simulink model "DZ1_2c"  (Simulink 7.5)
settings: Solver=ode45  StartTime=0.0  StopTime=100000  RelTol=1e-3
libraries: simulink x1
settings Model: Creator=Hrvoje  LastModifiedBy=Hrvoje

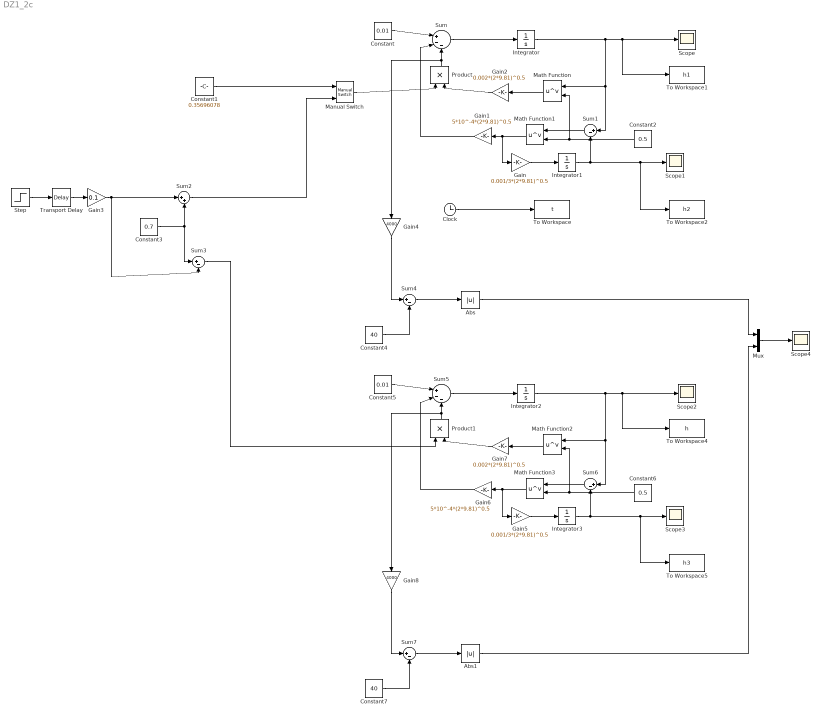
== system DZ1_2c ==
  Abs : Abs  OutDataType=fixdt(1, 16)  OutScaling=2^0
  Abs1 : Abs  OutDataType=fixdt(1, 16)  OutScaling=2^0
  Clock : Clock
      settings: Decimation=10
  Constant : Constant  Value=0.01  OutDataType=fixdt(1, 16)  OutScaling=2^0
  Constant1 : Constant  Value=0.35696078  OutDataType=fixdt(1, 16)  OutScaling=2^0
  Constant2 : Constant  Value=0.5  OutDataType=fixdt(1, 16)  OutScaling=2^0
  Constant3 : Constant  Value=0.7  OutDataType=fixdt(1, 16)  OutScaling=2^0
  Constant4 : Constant  Value=40  OutDataType=fixdt(1, 16)  OutScaling=2^0
  Constant5 : Constant  Value=0.01  OutDataType=fixdt(1, 16)  OutScaling=2^0
  Constant6 : Constant  Value=0.5  OutDataType=fixdt(1, 16)  OutScaling=2^0
  Constant7 : Constant  Value=40  OutDataType=fixdt(1, 16)  OutScaling=2^0
  Gain : Gain  Gain=0.001/3*(2*9.81)^0.5  ParameterDataType=fixdt(1, 16)  ParameterScaling=2^0  OutDataType=fixdt(1, 16)  OutScaling=2^0
  Gain1 : Gain  Gain=5*10^-4*(2*9.81)^0.5  ParameterDataType=fixdt(1, 16)  ParameterScaling=2^0  OutDataType=fixdt(1, 16)  OutScaling=2^0
  Gain2 : Gain  Gain=0.002*(2*9.81)^0.5  ParameterDataType=fixdt(1, 16)  ParameterScaling=2^0  OutDataType=fixdt(1, 16)  OutScaling=2^0
  Gain3 : Gain  Gain=0.1  ParameterDataType=fixdt(1, 16)  ParameterScaling=2^0  OutDataType=fixdt(1, 16)  OutScaling=2^0
  Gain4 : Gain  Gain=4000  ParameterDataType=fixdt(1, 16)  ParameterScaling=2^0  OutDataType=fixdt(1, 16)  OutScaling=2^0
  Gain5 : Gain  Gain=0.001/3*(2*9.81)^0.5  ParameterDataType=fixdt(1, 16)  ParameterScaling=2^0  OutDataType=fixdt(1, 16)  OutScaling=2^0
  Gain6 : Gain  Gain=5*10^-4*(2*9.81)^0.5  ParameterDataType=fixdt(1, 16)  ParameterScaling=2^0  OutDataType=fixdt(1, 16)  OutScaling=2^0
  Gain7 : Gain  Gain=0.002*(2*9.81)^0.5  ParameterDataType=fixdt(1, 16)  ParameterScaling=2^0  OutDataType=fixdt(1, 16)  OutScaling=2^0
  Gain8 : Gain  Gain=4000  ParameterDataType=fixdt(1, 16)  ParameterScaling=2^0  OutDataType=fixdt(1, 16)  OutScaling=2^0
  Integrator{,1..3} (4 alike) : Integrator  InitialCondition=2.6
  Manual Switch : simulink/Signal Routing/Manual Switch  SystemSampleTime=-1  sw=0  action=0  varsize=off
  Math Function{,1..3} (4 alike) : Math  Operator=pow  OutDataType=fixdt(1, 16)  OutScaling=2^0  SaturateOnIntegerOverflow=on
  Mux : Mux  Inputs=2
  Product : Product  OutDataType=fixdt(1, 16)  OutScaling=2^0  RndMeth=Zero
  Product1 : Product  OutDataType=fixdt(1, 16)  OutScaling=2^0  RndMeth=Zero
  Scope{,1..4} (5 alike) : Scope
      Scope2 settings: SaveName=ScopeData4
      Scope3 settings: SaveName=ScopeData5
      Scope4 settings: SaveName=ScopeData2
  Step : Step  SampleTime=0
  Sum : Sum  Inputs=|+--  OutDataType=fixdt(1, 16)  OutScaling=2^0
  Sum{1,3..4,6..7} (5 alike) : Sum  Inputs=|+-  OutDataType=fixdt(1, 16)  OutScaling=2^0
  Sum2 : Sum  Inputs=|++  OutDataType=fixdt(1, 16)  OutScaling=2^0
  Sum5 : Sum  Inputs=|+--  OutDataType=fixdt(1, 16)  OutScaling=2^0
  To Workspace : ToWorkspace  VariableName=t  SampleTime=-1  SaveFormat=Structure
  To Workspace1 : ToWorkspace  VariableName=h1  SampleTime=-1  SaveFormat=Structure
  To Workspace2 : ToWorkspace  VariableName=h2  SampleTime=-1  SaveFormat=Structure
  To Workspace4 : ToWorkspace  VariableName=h  SampleTime=-1  SaveFormat=Structure
  To Workspace5 : ToWorkspace  VariableName=h3  SampleTime=-1  SaveFormat=Structure
  Transport Delay : TransportDelay  DelayTime=1000
  wires:
  Constant/1 -> Sum/1
  Sum/1 -> Integrator/1
  Integrator/1 -> Scope/1, To Workspace1/1, Sum1/1, Math Function/1
  Integrator1/1 -> Sum1/2, Scope1/1, To Workspace2/1
  Gain/1 -> Integrator1/1
  Math Function1/1 -> Gain1/1, Gain/1
  Gain1/1 -> Sum/2
  Math Function/1 -> Gain2/1
  Gain2/1 -> Product/2
  Product/1 -> Sum/3, Gain4/1
  Clock/1 -> To Workspace/1
  Sum1/1 -> Math Function1/1
  Constant2/1 -> Math Function1/2, Math Function/2
  Manual Switch/1 -> Product/1
  Constant1/1 -> Manual Switch/1
  Step/1 -> Transport Delay/1
  Transport Delay/1 -> Gain3/1
  Gain3/1 -> Sum2/1, Sum3/2
  Constant3/1 -> Sum2/2, Sum3/1
  Sum2/1 -> Manual Switch/2
  Sum3/1 -> Product1/1
  Constant4/1 -> Sum4/2
  Gain4/1 -> Sum4/1
  Sum4/1 -> Abs/1
  Abs/1 -> Mux/1
  Constant5/1 -> Sum5/1
  Sum5/1 -> Integrator2/1
  Integrator2/1 -> Scope2/1, To Workspace4/1, Sum6/1, Math Function2/1
  Integrator3/1 -> Sum6/2, Scope3/1, To Workspace5/1
  Gain5/1 -> Integrator3/1
  Math Function3/1 -> Gain6/1, Gain5/1
  Gain6/1 -> Sum5/2
  Math Function2/1 -> Gain7/1
  Gain7/1 -> Product1/2
  Product1/1 -> Sum5/3, Gain8/1
  Sum6/1 -> Math Function3/1
  Constant6/1 -> Math Function3/2, Math Function2/2
  Constant7/1 -> Sum7/2
  Gain8/1 -> Sum7/1
  Sum7/1 -> Abs1/1
  Abs1/1 -> Mux/2
  Mux/1 -> Scope4/1
